simulink library "aerospace"  (R2022a)
settings: Solver=ode45  StartTime=0.0  StopTime=10.0  RelTol=1e-3
undefined symbols (not defined in the file or in its folder): __PRM__SERIALIZED__DATA__, BlockKeywords, convert, Math_Operations_Reshape_convert, Math_Operations_Reshape_reshape, pow
libraries: $bdroot x14
(part 1 of 2)
settings Model: Creator=The MathWorks, Inc.  LastModifiedBy=The MathWorks, Inc.
settings SolverCC: AlgebraicLoopSolver=TrustRegion
settings DataIOCC: LimitDataPoints=on  SaveFormat=Array  SignalLoggingSaveFormat=ModelDataLogs  ReturnWorkspaceOutputs=off
settings OptimizationCC: BlockReduction=off  BooleanDataType=off  ExpressionDepthLimit=2147483647  LifeSpan=inf
settings DebuggingCC: SaveWithParameterizedLinksMsg=none  SignalResolutionControl=TryResolveAllWithWarning  MultiTaskCondExecSysMsg=none  UnconnectedInputMsg=warning  UnconnectedOutputMsg=warning  UnconnectedLineMsg=warning  StateNameClashWarn=warning  SFUnexpectedBacktrackingDiag=warning  SFNoUnconditionalDefaultTransitionDiag=warning  SFExecutionAtInitializationDiag=none  SFMachineParentedDataDiag=warning  ArithmeticOperatorsInVariantConditions=warning
settings HardwareCC: ProdBitPerPointer=32  ProdBitPerSizeT=32  ProdBitPerPtrDiffT=32  ProdLargestAtomicFloat=None  ProdIntDivRoundTo=Undefined  ProdEndianess=Unspecified  ProdWordSize=32  ProdHWDeviceType=32-bit Generic  TargetUnknown=on
settings ModelReferenceCC: PropagateSignalLabelsOutOfModel=off
settings SFSimCC: SimUseLocalCustomCode=off  CustomCodeUndefinedFunction=UseInterfaceOnly
settings RTWCC: RTWUseLocalCustomCode=off
settings CodeAppCC: StateflowObjectComments=on
settings GRTTargetCC: TargetLangStandard=C89/C90 (ANSI)
settings ConfigComp: CovMetricSettings=d  CovSaveCumulativeToWorkspaceVar=on  CovSaveSingleToWorkspaceVar=on  CovExternalEMLEnable=off

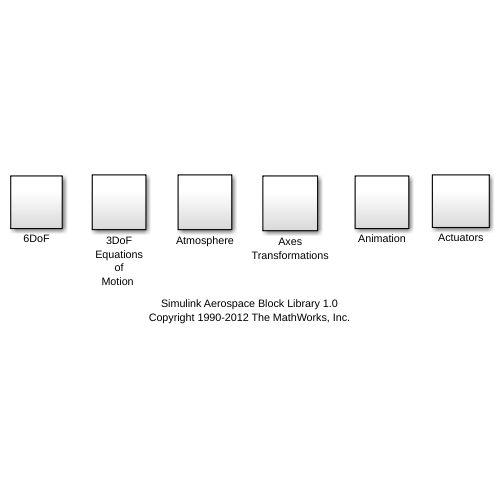
[thumbnail: Simulink's stored preview of the top-level diagram]
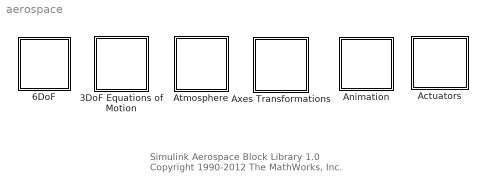
== system aerospace ==
  note: Simulink Aerospace Block Library 1.0
      | Copyright 1990-2012 The MathWorks, Inc.
  "3DoF Equations of Motion " : Subsystem
  6DoF : Subsystem
  Actuators : Subsystem
  Animation : Subsystem
  Atmosphere : Subsystem
  Axes Transformations : Subsystem

== system aerospace/3DoF Equations of Motion  ==
  " Equations of Motion (Body Axes)" : Subsystem  mask(3 DOF equations of motion){v_ini=100, theta_ini=0, alpha_ini=0, q_ini=0, pos_ini=[0 0], mass=1, Iyy=1, g=9.81}
      mask prompts: v_ini "Initial velocity [m/s]:"; theta_ini "Initial body attitude [rad]:"; alpha_ini "Initial incidence [rad]:"; q_ini "Initial body rotation rate [rad/sec]:"; pos_ini "Initial position (x z) [m]:"; mass "Mass [Kg]:"; Iyy "Inertia [Kg.m^2]:"; g "Acceleration due to gravity [m/s/s]:"
      mask help: Integrates the 3 degrees of freedom equations of motion to determine body position, velocity, attitude and related values.
      mask init:
      | U0 = v_ini*cos(alpha_ini);
      | w0 = v_ini*sin(alpha_ini);
      mask Help:
      | <p>This block models the 3 degrees of freedom equations of motion to determine body position, velocity, attitude and other related values.</p>
      | 
      | <p>A 3-down configuration for the body coordinates ( X axis pointing toward nose of body, and  Z axis pointing towards earth) is used in this block.</p>
      | 
      | <p>Gravitational force on the body is already accounted for in this block.</p>
      | 
      | <p>Some block outputs contain more than one signal as described below.</p>
      | 
      | <p><H4>Block  Inputs</H4>
      | <ul>
      |     <li>Forces on the body in X direction - Fx ( N )</li>
      |     <li>Forces on the body in Z direction - Fz ( N ) </li>
      |     <li>Moments on the body along Y direction - M ( N-m )</li>
      | </ul>
      | </p>
      | <p><H4>Block Outputs</H4>
      | <ul>
      |     <li>Pitch angle - Attitude ( radians )</li>
      |     <li>Pitch rate - q ( radians/sec )</li>
      |     <li>Pitch acceleration - qdot ( radians/sec^2 )</li>
      | </ul>
      | </p>
      | <p><H4>Block Vector Output - Xe, Ze </H4>
      | <ul>
      |     <li>Position in X direction in Earth coordinates - Xe ( m )</li>
      |     <li>Position in Z direction in Earth coordinates - Ze ( m )</li>
      | </ul>
      | </p>
      | <p><H4>Block Vector Output - U,w </H4>
      | <ul>
      |     <li>Translational velocity in X direction - U ( m/sec )</li>
      |     <li>Translational velocity in Z direction - w ( m/sec )</li>
      | </ul>
      | </p>
      | <p><H4>Block Vector Output - Ax, Az </H4>
      | <ul>
      |     <li>Acceleration in X direction due to body forces - Ax ( m/sec^2 )</li>
      |     <li>Acceleration in Z direction due to body forces - Az ( m/sec^2 )</li>
      | </ul>
      | </p>
  Incidence & Airspeed : Subsystem  mask(Incidence and Airspeed){}
      mask help: Calculates the angle between the body and the velocity vector (incidence) and the velocity magnitude from the components in body axes (U,w).
      mask Help:
      | <p>This block calculates the angle between the body and the velocity vector (incidence) and the velocity magnitude (airspeed) from the velocity components in body axes (U,w).</p>
      | 
      | <p> A 3-down configuration ( X axis pointing toward nose of body, and  Z axis pointing towards earth) is used in this block.</p>
      | 
      | <p>The block input contains more than one signal as described below.</p>
      | 
      | <p><H4>Block Vector  Input - U,w</H4>
      | <ul>
      |     <li>Translational velocity in X direction - U</li>
      |     <li>Translational velocity in Z direction - w</li>
      | </ul>
      | </p>
      | <p><H4>Block Outputs</H4>
      | <ul>
      |     <li>Incidence angle - alpha (radians)</li>
      |     <li>Airspeed - V</li>
      | </ul>
      | </p>

== system aerospace/6DoF ==
  Equations of Motion (Configurable Subsystem) : Subsystem  Variant=on  VariantControlMode=label  LabelModeActiveChoice=Euler Angles
      settings: AttributesFormatString=%<BlockChoice>
  Euler Angles : Subsystem  mask(6DoF Equations of Motion){xme_0=[0 0 0], Vm_0=[0 0 0], eul_0=[0 0 0], pm_0=[0 0 0], Mass=1.0, Inertia=eye(3)}
      mask prompts: xme_0 "Initial position in inertial axes [Xe,Ye,Ze]:"; Vm_0 "Initial velocity in body axes [U,v,w]:"; eul_0 "Initial Euler orientation [roll, pitch, yaw]:"; pm_0 "Initial body rotation rates [p,q,r]:"; Inertia "Inertia matrix:"
      mask help: Integrates the 6 degrees of freedom equations of motion using an euler angle representation for the orientation of the body in space.
      mask Help:
      | <p>This block models a 6 degrees of freedom equations of motion for a rigid body using an euler angle representation.</p>
      | 
      | <pThe block inputs and outputs contain more than one signal as described below.</p>
      | 
      | <p><H4>Block Vector  Input - Forces X Y Z</H4>
      | <ul>
      |     <li>Forces on the body in X direction - X </li>
      |     <li>Forces on the body in Y direction - Y </li>
      |     <li>Forces on the body in Z direction - Z </li>
      | </ul>
      | </p>
      | <p><H4>Block Vector  Input - Moments L M N</H4>
      | <ul>
      |     <li>Moments on the body along X direction - L </li>
      |     <li>Moments on the body along Y direction - M </li>
      |     <li>Moments on the body along Z direction - N </li>
      | </ul>
      | </p>
      | <p><H4>Block Vector Output - Ve </H4>
      | <ul>
      |     <li>Translational velocity in X direction in Inertial coordinates </li>
      |     <li>Translational velocity in Y direction in Inertial coordinates </li>
      |     <li>Translational velocity in Z direction in Inertial coordinates </li>
      | </ul>
      | </p>
      | <p><H4>Block Vector Output - Xe </H4>
      | <ul>
      |     <li>Position in X direction in Inertial coordinates - Xe </li>
      |     <li>Position in Y direction in Inertial coordinates - Ye </li>
      |     <li>Position in Z direction in Inertial coordinates - Ze </li>
      | </ul>
      | </p>
      | <p><H4>Block Vector Output - Euler </H4>
      | <ul>
      |     <li>Phi ( radians )</li>
      |     <li>Theta ( radians )</li>
      |     <li>Psi ( radians )</li>
      | </ul>
      | </p>
      | <p><H4>Block Vector Output - DMC </H4>
      | <ul>
      |     <li>3x3 Directional Cosine Matrix</li>
      | </ul>
      | </p>
      | <p><H4>Block Vector Output - Vb</H4>
      | <ul>
      |     <li>Translational velocity in X direction in Body coordinates </li>
      |     <li>Translational velocity in Y direction in Body coordinates </li>
      |     <li>Translational velocity in Z direction in Body coordinates </li>
      | </ul>
      | </p>
      | <p><H4>Block Vector Output - p, q, r</H4>
      | <ul>
      |     <li>Roll rate - p ( radians/sec )</li>
      |     <li>Pitch rate - q ( radians/sec )</li>
      |     <li>Yaw rate - r ( radians/sec )</li>
      | </ul>
      | </p>
      | <p><H4>Block Vector Output - pdot, qdot, rdot</H4>
      | <ul>
      |     <li>Roll acceleration - pdot ( radians/sec^2 )</li>
      |     <li>Pitch acceleration - qdot ( radians/sec^2 )</li>
      |     <li>Yaw acceleration - rdot ( radians/sec^2 )</li>
      | </ul>
      | </p>
      mask Display: disp('Euler\nAngles')
  Quaternions : Subsystem  mask(6DoF Equations of Motion){xme_0=[0 0 0], Vm_0=[0 0 0], eul_0=[0 0 0], pm_0=[0 0 0], Mass=1.0, Inertia=eye(3)}
      mask prompts: xme_0 "Initial position in inertial axes [Xe,Ye,Ze]:"; Vm_0 "Initial velocity in body axes [U,v,w]:"; eul_0 "Initial Euler orientation [roll, pitch, yaw]:"; pm_0 "Initial body rotation rates [p,q,r]:"; Inertia "Inertia matrix:"
      mask help: Integrates the 6 degrees of freedom equations of motion using a quaternion representation for the orientation of the body in space.
      mask init:
      | %%% factor used for quaternion calculation
      | k_quat=100;
      | 
      | %%% initial orientation of platform
      | ph=eul_0(1);
      | th=eul_0(2);
      | ps=eul_0(3);
      | e0_0 = cos(0.5*ps)*cos(0.5*th)*cos(0.5*ph) +sin(0.5*ps)*sin(0.5*th)*sin(0.5*ph);
      | e1_0 = cos(0.5*ps)*cos(0.5*th)*sin(0.5*ph) - sin(0.5*ps)*sin(0.5*th)*cos(0.5*ph);
      | e2_0 = cos(0.5*ps)*sin(0.5*th)*cos(0.5*ph) +sin(0.5*ps)*cos(0.5*th)*sin(0.5*ph);
      | e3_0 =-cos(0.5*ps)*sin(0.5*th)*sin(0.5*ph) +sin(0.5*ps)*cos(0.5*th)*cos(0.5*ph);
      mask Help:
      | <p>This block models a 6 degrees of freedom equations of motion for a rigid body using a quaternion representation.</p>
      | 
      | <pThe block inputs and outputs contain more than one signal as described below.</p>
      | 
      | <p><H4>Block Vector  Input - Forces X Y Z</H4>
      | <ul>
      |     <li>Forces on the body in X direction - X </li>
      |     <li>Forces on the body in Y direction - Y </li>
      |     <li>Forces on the body in Z direction - Z </li>
      | </ul>
      | </p>
      | <p><H4>Block Vector  Input - Moments L M N</H4>
      | <ul>
      |     <li>Moments on the body along X direction - L </li>
      |     <li>Moments on the body along Y direction - M </li>
      |     <li>Moments on the body along Z direction - N </li>
      | </ul>
      | </p>
      | <p><H4>Block Vector Output - Ve </H4>
      | <ul>
      |     <li>Translational velocity in X direction in Inertial coordinates </li>
      |     <li>Translational velocity in Y direction in Inertial coordinates </li>
      |     <li>Translational velocity in Z direction in Inertial coordinates </li>
      | </ul>
      | </p>
      | <p><H4>Block Vector Output - Xe </H4>
      | <ul>
      |     <li>Position in X direction in Inertial coordinates - Xe </li>
      |     <li>Position in Y direction in Inertial coordinates - Ye </li>
      |     <li>Position in Z direction in Inertial coordinates - Ze </li>
      | </ul>
      | </p>
      | <p><H4>Block Vector Output - Euler </H4>
      | <ul>
      |     <li>Phi ( radians )</li>
      |     <li>Theta ( radians )</li>
      |     <li>Psi ( radians )</li>
      | </ul>
      | </p>
      | <p><H4>Block Vector Output - DMC </H4>
      | <ul>
      |     <li>3x3 Directional Cosine Matrix</li>
      | </ul>
      | </p>
      | <p><H4>Block Vector Output - Vb</H4>
      | <ul>
      |     <li>Translational velocity in X direction in Body coordinates </li>
      |     <li>Translational velocity in Y direction in Body coordinates </li>
      |     <li>Translational velocity in Z direction in Body coordinates </li>
      | </ul>
      | </p>
      | <p><H4>Block Vector Output - p, q, r</H4>
      | <ul>
      |     <li>Roll rate - p ( radians/sec )</li>
      |     <li>Pitch rate - q ( radians/sec )</li>
      |     <li>Yaw rate - r ( radians/sec )</li>
      | </ul>
      | </p>
      | <p><H4>Block Vector Output - pdot, qdot, rdot</H4>
      | <ul>
      |     <li>Roll acceleration - pdot ( radians/sec^2 )</li>
      |     <li>Pitch acceleration - qdot ( radians/sec^2 )</li>
      |     <li>Yaw acceleration - rdot ( radians/sec^2 )</li>
      | </ul>
      | </p>
      mask Display: disp('Quaternions')

== system aerospace/Actuators ==
  2nd Order Non-linear Actuator : Subsystem  mask(Nonlinear 2nd order actuator model){wn_fin=150, z_fin=0.7, fin_max=20*pi/180, fin_min=-20*pi/180, fin_maxrate=500*pi/180, fin_act_0=0}
      mask prompts: wn_fin "Natural frequency:"; z_fin "Damping ratio:"; fin_max "Maximum deflection:"; fin_min "Minimum deflection:"; fin_maxrate "Maximum rate:"; fin_act_0 "Initial position:"
      mask help:
      | Implement a second-order actuator model with saturation and rate limits, where Ac_dem is the demanded actuator position and Ac_ac is the actual actuator position.
      |
      | Input, output, minimum deflection, maximum deflection, and initial position are in the same position units defined by the input signal.  Maximum rate has the units of position/seconds.
      mask Help:
      | <p>This block contains a model of a second order non-linear actuator.  In addition to setting actuator initial position, damping ratio and natural frequency, block parameters allow fin deflection maximum and minimum limits to be set and a rate limit to be set for the actuator.</p>
      | 
      | <p><H4>Block Input</H4>
      | <ul>
      | <li>Commanded actuator position</li>
      | </ul>
      | </p>
      | 
      | <p><H4>Block Output</H4>
      | <ul>
      | <li>Actual actuator position</li>
      | </ul>
      | </p>
  2nd Order linear Actuator : Subsystem  mask(Linear 2nd order actuator model.){wn_fin=150, z_fin=0.7, fin_act_0=0}
      mask prompts: wn_fin "Natural frequency:"; z_fin "Damping ratio:"; fin_act_0 "Initial position:"
      mask help:
      | Implement a second-order actuator model where Ac_dem is the demanded actuator position and Ac_ac is the actual actuator position.
      |
      | Input, output, and initial position are in the same position units defined by the input signal.
      mask Help:
      | <p>This block contains a model of a second order linear actuator.  Block parameters allow initial position, damping ratio and natural frequency to be set for the  actuator.</p>
      | 
      | <p><H4>Block Input</H4>
      | <ul>
      | <li>Commanded actuator position</li>
      | </ul>
      | </p>
      | 
      | <p><H4>Block Output</H4>
      | <ul>
      | <li>Actual actuator position</li>
      | </ul>
      | </p>

== system aerospace/Animation ==
  3DoF Animation : Subsystem  mask(3DoF Animation){u1=[0 5000 -2000 2000 -5050 -3050], u2=0.05, u3=1, u5=Fixed position, u6=[2000 500 -3150], u7=10, u8=on}
      mask prompts: u1 "Axes limits [xmin xmax ymin ymax zmin zmax]:"; u2 "Time interval between updates:"; u3 "Size of craft displayed:"; u5 "Enter view:"; u6 "Position of camera [xc yc zc]:"; u7 "View angle:"; u8 "Enable animation"
      mask help:
      | Create a 3-D animated view of a three-degrees-of-freedom craft and its target, where X and Z target position (TargetPos), X and Z craft position (Xe,Ze), and craft attitude are inputs.
      |
      | Display parameters are in the same units of length as the input parameters.
      mask init:
      | Config.axes = u1;
      | Config.update = u2;
      | Config.craft = u3;
      | Config.camera_view = u5;
      | Config.camera_pos = u6;
      | Config.view = u7;
      | Config.Animenable = u8;
      mask Help:
      | <p>This block generates a 3 dimensional display of a 3 degrees of freedom trajectory, with the craft's orientation displayed during flight from a viewer position, including a target displayed for the object.  See also: Simulink model 'guidance'.</p>
      | 
      | <p><H4>Block Inputs</H4>
      | <ul>
      | <li>Target position  - [ X, Y, Z ] coordinates
      | <li>[Xe, Ze] - object's range and altitude
      | <li>Attitude - object's pitch angle
      | </ul></p>
      mask TypeOptions u5: Fixed position | Cockpit | Fly alongside
  6DoF Animation : Subsystem  mask(6DoF Animation){u1=[0 4000 -2000 2000 -5000 -3000], u2=0.1, u3=1.0, u4=[4000 0 -5000], u5=Fixed position, u6=[2000 500 -3150], u7=10, u8=on}
      mask prompts: u1 "Axes limits [xmin xmax ymin ymax zmin zmax]:"; u2 "Time interval between updates:"; u3 "Size of craft displayed:"; u4 "Static object position [xp yp zp]:"; u5 "Enter view:"; u6 "Position of camera [xc yc zc]:"; u7 "View angle:"; u8 "Enable animation"
      mask help:
      | Create a 3-D animated view of a six-degrees-of-freedom craft, where X, Y, and Z craft position (Position) and craft Euler angles (Euler) are inputs.
      |
      | Display parameters are in the same units of length as the input parameters.
      mask init:
      | Config.axes = u1;
      | Config.update = u2;
      | Config.craft = u3;
      | Config.target = u4;
      | Config.camera_view = u5;
      | Config.camera_pos = u6;
      | Config.view = u7;
      | Config.Animenable = u8;
      mask Help:
      | <p>This block generates a 3 dimensional display of a simulation trajectory, with the craft orientation displayed during flight</p>
      | 
      | <p>There are two inputs to this block, Position and Euler.  These inputs contain more than one signal as described below.</p>
      | 
      | <p><H4>Block Vector Input - Position</H4>
      | <ul>
      | <li>X Position</li>
      | <li>Y Position</li>
      | <li>Z Position</li>
      | </ul>
      | </p>
      | 
      | <p><H4>Block Vector Input - Euler</H4>
      |     <ul>
      |     <li>Roll Attitude</li>
      |     <li>Pitch Attitude</li>
      |     <li>Yaw Attitude</li>
      |    </ul>
      |    </p>
      mask TypeOptions u5: Fixed position | Cockpit | Fly alongside

== system aerospace/Atmosphere ==
  Atmosphere model : Subsystem  mask(Atmosphere Model){}
      mask help: Compute International Standard Atmosphere (ISA) model for altitudes between 0 Km and 20 Km.
      mask init:
      | g=9.80665; % m/s
      | gamma = 1.4;
      | R = 287.0531; %J/Kg/K
      | L = 0.0065; % K/m
      | h_trop = 11000; % m
      | rho0 = 1.225; %Kg/m^3
      | P0 = 101325; % Pa
      | T0 = 288.15; % K
      mask Help:
      | <p>This block contains the International Standard Atmosphere (ISA) model for altitudes between 0 and 20 Km.  If the height input is greater than 20 Km, the height will be limited to 20 Km.</p>
      | 
      | <p><H4>Block Input</H4>
      | <ul>
      |     <li>Height - Altitude in meters</li>
      | </ul>
      | </p>
      | <p><H4>Block Outputs</H4>
      | <ul>
      |     <li>Temperature - in degree Kelvin</li>
      |     <li>Speed of Sound - in meters/second</li>
      |     <li>Air Pressure - in Pascals</li>
      |     <li>Air Density - in kilograms/meter</li>
      | </ul>
      | </p>

== system aerospace/Axes Transformations ==
  3x3 cross product : Subsystem  mask(Cross Product){}
      mask help: Calculates the cross product of two 3x1 vectors.
      mask Help:
      | <p>This block calculates the cross product of two 3x1 vectors, ie.</p>
      | 
      | <ul>C(1) = A(2)*B(3) - A(3)*B(2)</ul>
      | <ul>C(2) = A(3)*B(1) - A(1)*B(3)</ul>
      | <ul>C(3) = A(1)*B(2) - A(2)*B(1)</ul>
      | 
      | <p>The block inputs and output contain more than one signal as described below.</p>
      | 
      | <p><H4>Block Vector Input 1 - A</H4>
      | <ul>
      | <li>A(1)</li>
      | <li>A(2)</li>
      | <li>A(3)</li>
      | </ul>
      | </p>
      | 
      | <p><H4>Block Vector Input 2 - B</H4>
      | <ul>
      | <li>B(1)</li>
      | <li>B(2)</li>
      | <li>B(3)</li>
      | </ul>
      | </p>
      | 
      | <p><H4>Block Vector Output - Cross Product (AxB)</H4>
      | <ul>
      | <li>C(1)</li>
      | <li>C(2)</li>
      | <li>C(3)</li>
      | </ul>
      | </p>
      mask Display: disp('Cross\nProduct')
  Direction Cosine Matrix from Euler Angles : Subsystem  mask(Direction Cosine Matrix){}
      mask help: Determines the 3x3 Direction Cosine Matrix (DCM) from an euler orientation (roll, pitch, yaw). The outputted DCM transforms vectors from inertial axes to body axes.
      mask Help:
      | <p>This block determines the 3x3 Direction Cosine Matrix (DCM) from a 3x1 euler orientation. The outputted DCM transforms vectors from inertial axes to body axes.</p>
      | 
      | <p>The block input and output contain more than one signal as described below.</p>
      | 
      | <p><H4>Block Vector Input - Euler </H4>
      |     <ul>
      |     <li>Roll Attitude</li>
      |     <li>Pitch Attitude</li>
      |     <li>Yaw Attitude</li>
      |    </ul>
      |    </p>
      | 
      | <p><H4>Block Matrix Output - Direction Cosine Matrix </H4>
      |     <ul>
      |    </ul>
      |    </p>
      mask Display: disp('axis')
  Direction Cosine Matrix from quaternions : Subsystem  mask(Direction Cosine Matrix){}
      mask help: Determines the 3x3 Direction Cosine Matrix (DCM) from a 4x1 quaternion orientation vector. The outputted DCM transforms vectors from inertial axes to body axes.
      mask Help:
      | <p>This block determines the 3x3 Direction Cosine Matrix (DCM) from a 4x1 quaternion orientation vector. The outputted DCM transforms vectors from inertial axes to body axes.</p>
      | 
      | <p>The block input and output contain more than one signal as described below.</p>
      | 
      | <p><H4>Block Vector Input - Quaternion</H4>
      | <ul>
      | <li>q0</li>
      | <li>q1</li>
      | <li>q2</li>
      | <li>q3</li>
      | </ul>
      | </p>
      | 
      | <p><H4>Block Matrix Output - Direction Cosine Matrix  </H4>
      |     <ul>
      |    </ul>
      |    </p>
      mask Display: disp('axis')
  Euler angles from quaternions : Subsystem  mask(Euler angles){}
      mask help: Calculates Euler angles (Roll, Pitch, Yaw) from Quaternions (q0,q1,q2,q3)
      mask Help:
      | <p>This block calculates a 3x1 euler orientation vector from a 4x1 quaternion orientation vector.</p>
      | 
      | <p>The block input and output contain more than one signal as described below.</p>
      | 
      | <p><H4>Block Vector Input - Quaternion</H4>
      | <ul>
      | <li>q0</li>
      | <li>q1</li>
      | <li>q2</li>
      | <li>q3</li>
      | </ul>
      | </p>
      | 
      | <p><H4>Block Vector Output - Euler </H4>
      |     <ul>
      |     <li>Roll Attitude</li>
      |     <li>Pitch Attitude</li>
      |     <li>Yaw Attitude</li>
      |    </ul>
      |    </p>
      mask Display: disp('angles')

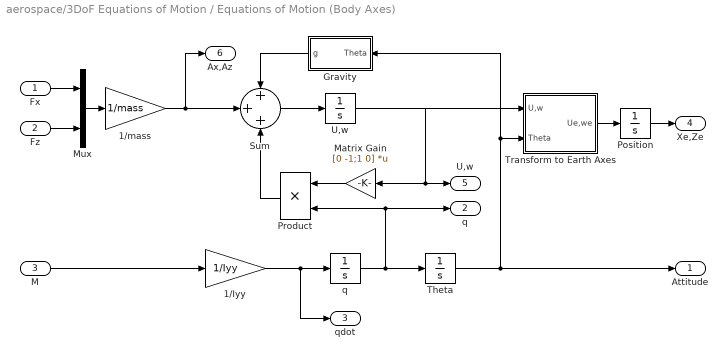
== system aerospace/3DoF Equations of Motion / Equations of Motion (Body Axes) ==
  Fx : Inport
  Fz : Inport  Port=2
  M : Inport  Port=3
  1/Iyy : Gain  Gain=1/Iyy  SaturateOnIntegerOverflow=on  OutDataTypeStr=Inherit: Same as input  ParamDataTypeStr=Inherit: Same as input
  1/mass : Gain  Gain=1/mass  SaturateOnIntegerOverflow=on  OutDataTypeStr=Inherit: Same as input  ParamDataTypeStr=Inherit: Same as input
  Gravity : Subsystem
  Matrix Gain : Gain  Gain=[0 -1;1 0]  Multiplication=Matrix(K*u)  SaturateOnIntegerOverflow=on  OutDataTypeStr=Inherit: Same as input  ParamDataTypeStr=Inherit: Same as input
  Mux : Mux  Inputs=2
  Position : Integrator  InitialCondition=pos_ini
  Product : Product  InputSameDT=on  RndMeth=Zero  SaturateOnIntegerOverflow=on  OutDataTypeStr=Inherit: Same as first input
  Sum : Sum  Inputs=+++  InputSameDT=on  SaturateOnIntegerOverflow=on  OutDataTypeStr=Inherit: Same as first input
  Theta : Integrator  InitialCondition=theta_ini
  Transform to Earth Axes : Subsystem
  U,w : Integrator  InitialCondition=[U0 w0]
  q : Integrator  InitialCondition=q_ini
  Attitude : Outport  InitialOutput=0  VectorParamsAs1DForOutWhenUnconnected=off
  "q " : Outport  Port=2  InitialOutput=0  VectorParamsAs1DForOutWhenUnconnected=off
  qdot : Outport  Port=3  InitialOutput=0  VectorParamsAs1DForOutWhenUnconnected=off
  Xe,Ze : Outport  Port=4  InitialOutput=0  VectorParamsAs1DForOutWhenUnconnected=off
  "U,w " : Outport  Port=5  InitialOutput=0  VectorParamsAs1DForOutWhenUnconnected=off
  Ax,Az : Outport  Port=6  InitialOutput=0  VectorParamsAs1DForOutWhenUnconnected=off
  wires:
  Sum/1 -> U,w/1
  q/1 -> Theta/1, "q "/1, Product/2
  M/1 -> 1/Iyy/1
  1/Iyy/1 -> q/1, qdot/1
  Theta/1 -> Attitude/1, Transform to Earth Axes/2(Theta), Gravity/1(Theta)
  U,w/1 -> Matrix Gain/1, Transform to Earth Axes/1(U,w), "U,w "/1
  Position/1 -> Xe,Ze/1
  Matrix Gain/1 -> Product/1
  Transform to Earth Axes/1(Ue,we) -> Position/1
  Fx/1 -> Mux/1
  Fz/1 -> Mux/2
  Mux/1 -> 1/mass/1
  Product/1 -> Sum/3
  1/mass/1 -> Ax,Az/1, Sum/2
  Gravity/1(g) -> Sum/1

== system aerospace/3DoF Equations of Motion /Incidence & Airspeed ==
  U,w : Inport
  Incidence : Fcn  Expr=atan2(u(2),u(1))
  Velocity : Fcn  Expr=sqrt(u(1)*u(1)+u(2)*u(2))
  Alpha : Outport  InitialOutput=0  VectorParamsAs1DForOutWhenUnconnected=off
  V : Outport  Port=2  InitialOutput=0  VectorParamsAs1DForOutWhenUnconnected=off
  wires:
  Velocity/1 -> V/1
  Incidence/1 -> Alpha/1
  U,w/1 -> Velocity/1, Incidence/1

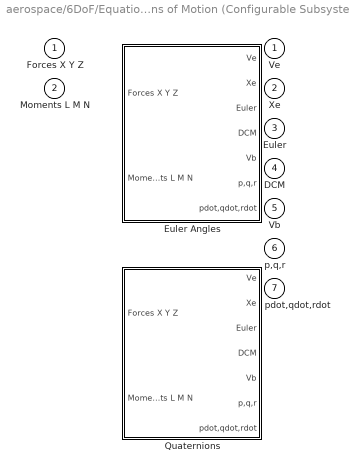
== system aerospace/6DoF/Equations of Motion (Configurable Subsystem) ==
  Forces X Y Z : Inport
  Moments L M N : Inport  Port=2
  Euler Angles : Subsystem  VariantControl=Euler Angles  mask(6DoF Equations of Motion){xme_0=[0 0 0], Vm_0=[0 0 0], eul_0=[0 0 0], pm_0=[0 0 0], Mass=1.0, Inertia=eye(3)}
      mask prompts: xme_0 "Initial position in inertial axes [Xe,Ye,Ze]:"; Vm_0 "Initial velocity in body axes [U,v,w]:"; eul_0 "Initial Euler orientation [roll, pitch, yaw]:"; pm_0 "Initial body rotation rates [p,q,r]:"; Inertia "Inertia matrix:"
      mask help: Integrates the 6 degrees of freedom equations of motion using an euler angle representation for the orientation of the body in space.
      mask Help:
      | <p>This block models a 6 degrees of freedom equations of motion for a rigid body using an euler angle representation.</p>
      | 
      | <pThe block inputs and outputs contain more than one signal as described below.</p>
      | 
      | <p><H4>Block Vector  Input - Forces X Y Z</H4>
      | <ul>
      |     <li>Forces on the body in X direction - X </li>
      |     <li>Forces on the body in Y direction - Y </li>
      |     <li>Forces on the body in Z direction - Z </li>
      | </ul>
      | </p>
      | <p><H4>Block Vector  Input - Moments L M N</H4>
      | <ul>
      |     <li>Moments on the body along X direction - L </li>
      |     <li>Moments on the body along Y direction - M </li>
      |     <li>Moments on the body along Z direction - N </li>
      | </ul>
      | </p>
      | <p><H4>Block Vector Output - Ve </H4>
      | <ul>
      |     <li>Translational velocity in X direction in Inertial coordinates </li>
      |     <li>Translational velocity in Y direction in Inertial coordinates </li>
      |     <li>Translational velocity in Z direction in Inertial coordinates </li>
      | </ul>
      | </p>
      | <p><H4>Block Vector Output - Xe </H4>
      | <ul>
      |     <li>Position in X direction in Inertial coordinates - Xe </li>
      |     <li>Position in Y direction in Inertial coordinates - Ye </li>
      |     <li>Position in Z direction in Inertial coordinates - Ze </li>
      | </ul>
      | </p>
      | <p><H4>Block Vector Output - Euler </H4>
      | <ul>
      |     <li>Phi ( radians )</li>
      |     <li>Theta ( radians )</li>
      |     <li>Psi ( radians )</li>
      | </ul>
      | </p>
      | <p><H4>Block Vector Output - DMC </H4>
      | <ul>
      |     <li>3x3 Directional Cosine Matrix</li>
      | </ul>
      | </p>
      | <p><H4>Block Vector Output - Vb</H4>
      | <ul>
      |     <li>Translational velocity in X direction in Body coordinates </li>
      |     <li>Translational velocity in Y direction in Body coordinates </li>
      |     <li>Translational velocity in Z direction in Body coordinates </li>
      | </ul>
      | </p>
      | <p><H4>Block Vector Output - p, q, r</H4>
      | <ul>
      |     <li>Roll rate - p ( radians/sec )</li>
      |     <li>Pitch rate - q ( radians/sec )</li>
      |     <li>Yaw rate - r ( radians/sec )</li>
      | </ul>
      | </p>
      | <p><H4>Block Vector Output - pdot, qdot, rdot</H4>
      | <ul>
      |     <li>Roll acceleration - pdot ( radians/sec^2 )</li>
      |     <li>Pitch acceleration - qdot ( radians/sec^2 )</li>
      |     <li>Yaw acceleration - rdot ( radians/sec^2 )</li>
      | </ul>
      | </p>
      mask Display: disp('Euler\nAngles')
  Quaternions : Subsystem  VariantControl=Quaternions  mask(6DoF Equations of Motion){xme_0=[0 0 0], Vm_0=[0 0 0], eul_0=[0 0 0], pm_0=[0 0 0], Mass=1.0, Inertia=eye(3)}
      mask prompts: xme_0 "Initial position in inertial axes [Xe,Ye,Ze]:"; Vm_0 "Initial velocity in body axes [U,v,w]:"; eul_0 "Initial Euler orientation [roll, pitch, yaw]:"; pm_0 "Initial body rotation rates [p,q,r]:"; Inertia "Inertia matrix:"
      mask help: Integrates the 6 degrees of freedom equations of motion using a quaternion representation for the orientation of the body in space.
      mask init: same as aerospace/6DoF/Quaternions
      mask Help:
      | <p>This block models a 6 degrees of freedom equations of motion for a rigid body using a quaternion representation.</p>
      | 
      | <pThe block inputs and outputs contain more than one signal as described below.</p>
      | 
      | <p><H4>Block Vector  Input - Forces X Y Z</H4>
      | <ul>
      |     <li>Forces on the body in X direction - X </li>
      |     <li>Forces on the body in Y direction - Y </li>
      |     <li>Forces on the body in Z direction - Z </li>
      | </ul>
      | </p>
      | <p><H4>Block Vector  Input - Moments L M N</H4>
      | <ul>
      |     <li>Moments on the body along X direction - L </li>
      |     <li>Moments on the body along Y direction - M </li>
      |     <li>Moments on the body along Z direction - N </li>
      | </ul>
      | </p>
      | <p><H4>Block Vector Output - Ve </H4>
      | <ul>
      |     <li>Translational velocity in X direction in Inertial coordinates </li>
      |     <li>Translational velocity in Y direction in Inertial coordinates </li>
      |     <li>Translational velocity in Z direction in Inertial coordinates </li>
      | </ul>
      | </p>
      | <p><H4>Block Vector Output - Xe </H4>
      | <ul>
      |     <li>Position in X direction in Inertial coordinates - Xe </li>
      |     <li>Position in Y direction in Inertial coordinates - Ye </li>
      |     <li>Position in Z direction in Inertial coordinates - Ze </li>
      | </ul>
      | </p>
      | <p><H4>Block Vector Output - Euler </H4>
      | <ul>
      |     <li>Phi ( radians )</li>
      |     <li>Theta ( radians )</li>
      |     <li>Psi ( radians )</li>
      | </ul>
      | </p>
      | <p><H4>Block Vector Output - DMC </H4>
      | <ul>
      |     <li>3x3 Directional Cosine Matrix</li>
      | </ul>
      | </p>
      | <p><H4>Block Vector Output - Vb</H4>
      | <ul>
      |     <li>Translational velocity in X direction in Body coordinates </li>
      |     <li>Translational velocity in Y direction in Body coordinates </li>
      |     <li>Translational velocity in Z direction in Body coordinates </li>
      | </ul>
      | </p>
      | <p><H4>Block Vector Output - p, q, r</H4>
      | <ul>
      |     <li>Roll rate - p ( radians/sec )</li>
      |     <li>Pitch rate - q ( radians/sec )</li>
      |     <li>Yaw rate - r ( radians/sec )</li>
      | </ul>
      | </p>
      | <p><H4>Block Vector Output - pdot, qdot, rdot</H4>
      | <ul>
      |     <li>Roll acceleration - pdot ( radians/sec^2 )</li>
      |     <li>Pitch acceleration - qdot ( radians/sec^2 )</li>
      |     <li>Yaw acceleration - rdot ( radians/sec^2 )</li>
      | </ul>
      | </p>
      mask Display: disp('Quaternions')
  Ve : Outport  VectorParamsAs1DForOutWhenUnconnected=off
  Xe : Outport  Port=2  VectorParamsAs1DForOutWhenUnconnected=off
  Euler : Outport  Port=3  VectorParamsAs1DForOutWhenUnconnected=off
  DCM : Outport  Port=4  VectorParamsAs1DForOutWhenUnconnected=off
  Vb : Outport  Port=5  VectorParamsAs1DForOutWhenUnconnected=off
  p,q,r : Outport  Port=6  VectorParamsAs1DForOutWhenUnconnected=off
  pdot,qdot,rdot : Outport  Port=7  VectorParamsAs1DForOutWhenUnconnected=off

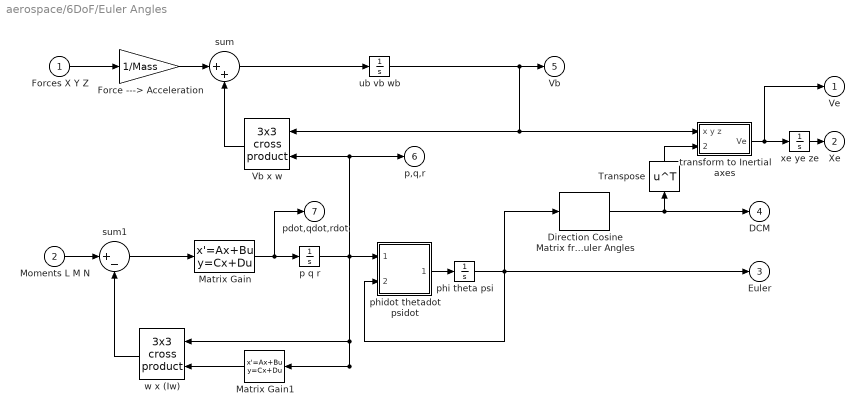
== system aerospace/6DoF/Euler Angles ==
  Forces X Y Z : Inport
  Moments L M N : Inport  Port=2
  Direction Cosine Matrix from Euler Angles : $bdroot/Axes Transformations/Direction Cosine Matrix from Euler Angles
  Force ---> Acceleration : Gain  Gain=1/Mass  SaturateOnIntegerOverflow=on  OutDataTypeStr=Inherit: Same as input  ParamDataTypeStr=Inherit: Same as input
  Matrix Gain : StateSpace  A=[]  B=[]  C=[]  D=K  InitialCondition=0  mask(Matrix Gain){K=inv(Inertia)}
      mask prompts: K "Gain matrix:"
      mask help: Matrix Gain.
      mask Help: Multiplies input vector by entered matrix to produce output vector (y=Au).
      mask Display: disp('Inertia^(-1)')
  Matrix Gain1 : StateSpace  A=[]  B=[]  C=[]  D=K  InitialCondition=0  mask(Matrix Gain){K=Inertia}
      mask prompts: K "Gain matrix:"
      mask help: Matrix Gain.
      mask Help: Multiplies input vector by entered matrix to produce output vector (y=Au).
      mask Display: disp('Inertia')
  Transpose : Math  Operator=transpose  SignedPower=on
  Vb x w : $bdroot/Axes Transformations/3x3 cross product
  p q r : Integrator  InitialCondition=pm_0
  phi theta psi : Integrator  InitialCondition=eul_0
  phidot thetadot psidot : Subsystem
  sum : Sum  Inputs=|++  InputSameDT=on  SaturateOnIntegerOverflow=on  OutDataTypeStr=Inherit: Same as first input
  sum1 : Sum  Inputs=|+-  InputSameDT=on  SaturateOnIntegerOverflow=on  OutDataTypeStr=Inherit: Same as first input
  "transform to Inertial axes " : Subsystem  mask(Vector Transformation){}
      mask Display: disp('L_EB')
  ub vb wb : Integrator  InitialCondition=Vm_0
  w x (Iw) : $bdroot/Axes Transformations/3x3 cross product
  xe ye ze : Integrator  InitialCondition=xme_0
  Ve : Outport  InitialOutput=0  VectorParamsAs1DForOutWhenUnconnected=off
  Xe : Outport  Port=2  InitialOutput=0  VectorParamsAs1DForOutWhenUnconnected=off
  Euler : Outport  Port=3  InitialOutput=0  VectorParamsAs1DForOutWhenUnconnected=off
  DCM : Outport  Port=4  InitialOutput=0  VectorParamsAs1DForOutWhenUnconnected=off
  Vb : Outport  Port=5  InitialOutput=0  VectorParamsAs1DForOutWhenUnconnected=off
  p,q,r : Outport  Port=6  InitialOutput=0  VectorParamsAs1DForOutWhenUnconnected=off
  pdot,qdot,rdot : Outport  Port=7  InitialOutput=0  VectorParamsAs1DForOutWhenUnconnected=off
  wires:
  phidot thetadot psidot/1(phidot thetadot psi) -> phi theta psi/1
  phi theta psi/1 -> Euler/1, phidot thetadot psidot/2(phi theta psi), Direction Cosine Matrix from Euler Angles/1
  ub vb wb/1 -> Vb/1, Vb x w/1, "transform to Inertial axes "/1(x y z)
  sum/1 -> ub vb wb/1
  xe ye ze/1 -> Xe/1
  "transform to Inertial axes "/1(Ve) -> xe ye ze/1, Ve/1
  p q r/1 -> Vb x w/2, p,q,r/1, Matrix Gain1/1, phidot thetadot psidot/1(p q r), w x (Iw)/1
  sum1/1 -> Matrix Gain/1
  Moments L M N/1 -> sum1/1
  Matrix Gain1/1 -> w x (Iw)/2
  w x (Iw)/1 -> sum1/2
  Matrix Gain/1 -> p q r/1, pdot,qdot,rdot/1
  Forces X Y Z/1 -> Force ---> Acceleration/1
  Vb x w/1 -> sum/2
  Force ---> Acceleration/1 -> sum/1
  Direction Cosine Matrix from Euler Angles/1 -> Transpose/1, DCM/1
  Transpose/1 -> "transform to Inertial axes "/2(transform coefficients)

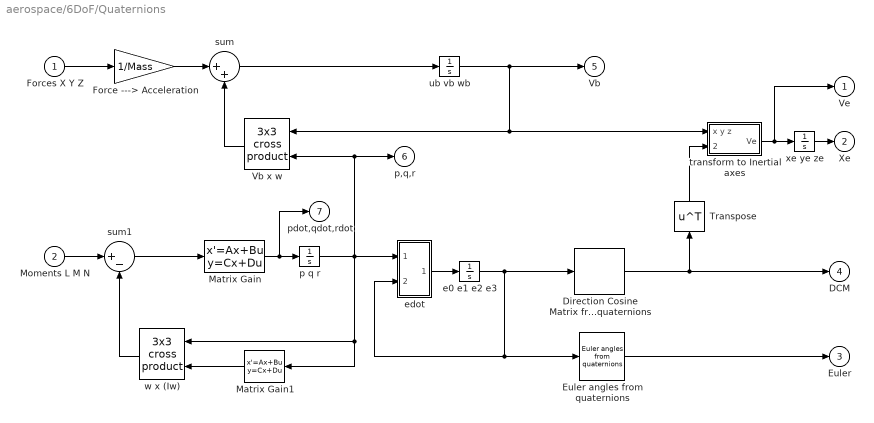
== system aerospace/6DoF/Quaternions ==
  Forces X Y Z : Inport
  Moments L M N : Inport  Port=2
  Direction Cosine Matrix from quaternions : $bdroot/Axes Transformations/Direction Cosine Matrix from quaternions
  Euler angles from quaternions : $bdroot/Axes Transformations/Euler angles from quaternions
  Force ---> Acceleration : Gain  Gain=1/Mass  SaturateOnIntegerOverflow=on  OutDataTypeStr=Inherit: Same as input  ParamDataTypeStr=Inherit: Same as input
  Matrix Gain : StateSpace  A=[]  B=[]  C=[]  D=K  InitialCondition=0  mask(Matrix Gain){K=inv(Inertia)}
      mask prompts: K "Gain matrix:"
      mask help: Matrix Gain.
      mask Help: Multiplies input vector by entered matrix to produce output vector (y=Au).
      mask Display: disp('Inertia^(-1)')
  Matrix Gain1 : StateSpace  A=[]  B=[]  C=[]  D=K  InitialCondition=0  mask(Matrix Gain){K=Inertia}
      mask prompts: K "Gain matrix:"
      mask help: Matrix Gain.
      mask Help: Multiplies input vector by entered matrix to produce output vector (y=Au).
      mask Display: disp('Inertia')
  Transpose : Math  Operator=transpose  SignedPower=on
  Vb x w : $bdroot/Axes Transformations/3x3 cross product
  e0 e1 e2 e3 : Integrator  InitialCondition=[e0_0 e1_0 e2_0 e3_0]
  edot : Subsystem
  p q r : Integrator  InitialCondition=pm_0
  sum : Sum  Inputs=|++  InputSameDT=on  SaturateOnIntegerOverflow=on  OutDataTypeStr=Inherit: Same as first input
  sum1 : Sum  Inputs=|+-  InputSameDT=on  SaturateOnIntegerOverflow=on  OutDataTypeStr=Inherit: Same as first input
  "transform to Inertial axes " : Subsystem  mask(Vector Transformation){}
      mask Display: disp('L_EB')
  ub vb wb : Integrator  InitialCondition=Vm_0
  w x (Iw) : $bdroot/Axes Transformations/3x3 cross product
  xe ye ze : Integrator  InitialCondition=xme_0
  Ve : Outport  InitialOutput=0  VectorParamsAs1DForOutWhenUnconnected=off
  Xe : Outport  Port=2  InitialOutput=0  VectorParamsAs1DForOutWhenUnconnected=off
  Euler : Outport  Port=3  InitialOutput=0  VectorParamsAs1DForOutWhenUnconnected=off
  DCM : Outport  Port=4  InitialOutput=0  VectorParamsAs1DForOutWhenUnconnected=off
  Vb : Outport  Port=5  InitialOutput=0  VectorParamsAs1DForOutWhenUnconnected=off
  p,q,r : Outport  Port=6  InitialOutput=0  VectorParamsAs1DForOutWhenUnconnected=off
  pdot,qdot,rdot : Outport  Port=7  InitialOutput=0  VectorParamsAs1DForOutWhenUnconnected=off
  wires:
  p q r/1 -> edot/1(in_1), Vb x w/2, p,q,r/1, Matrix Gain1/1, w x (Iw)/1
  sum1/1 -> Matrix Gain/1
  Moments L M N/1 -> sum1/1
  Matrix Gain1/1 -> w x (Iw)/2
  w x (Iw)/1 -> sum1/2
  edot/1(out_1) -> e0 e1 e2 e3/1
  e0 e1 e2 e3/1 -> Direction Cosine Matrix from quaternions/1, Euler angles from quaternions/1, edot/2(in_2)
  Euler angles from quaternions/1 -> Euler/1
  Matrix Gain/1 -> p q r/1, pdot,qdot,rdot/1
  Direction Cosine Matrix from quaternions/1 -> Transpose/1, DCM/1
  ub vb wb/1 -> Vb/1, Vb x w/1, "transform to Inertial axes "/1(x y z)
  Forces X Y Z/1 -> Force ---> Acceleration/1
  Vb x w/1 -> sum/2
  sum/1 -> ub vb wb/1
  Force ---> Acceleration/1 -> sum/1
  xe ye ze/1 -> Xe/1
  "transform to Inertial axes "/1(Ve) -> xe ye ze/1, Ve/1
  Transpose/1 -> "transform to Inertial axes "/2(transform coefficients)

== system aerospace/Actuators/2nd Order Non-linear Actuator ==
  Ac_dem : Inport
  2*zeta * wn : Gain  Gain=2.0 * z_fin* wn_fin  SaturateOnIntegerOverflow=on  OutDataTypeStr=Inherit: Same as input  ParamDataTypeStr=Inherit: Same as input
  Demand limits : Saturate  UpperLimit=fin_max  LowerLimit=fin_min
  Limited Deflection : Integrator  InitialCondition=fin_act_0  LimitOutput=on  UpperSaturationLimit=fin_max  LowerSaturationLimit=fin_min
  Servo rate : Integrator
  Sum2 : Sum  Inputs=|+-  InputSameDT=on  SaturateOnIntegerOverflow=on  OutDataTypeStr=Inherit: Same as first input
  Sum3 : Sum  Inputs=|+-  InputSameDT=on  SaturateOnIntegerOverflow=on  OutDataTypeStr=Inherit: Same as first input
  rate limit*2*zeta/wn : Saturate  UpperLimit=fin_maxrate*2*z_fin/wn_fin  LowerLimit=-fin_maxrate*2*z_fin/wn_fin
  wn^2 : Gain  Gain=wn_fin* wn_fin  SaturateOnIntegerOverflow=on  OutDataTypeStr=Inherit: Same as input  ParamDataTypeStr=Inherit: Same as input
  Ac_ac : Outport  InitialOutput=0  VectorParamsAs1DForOutWhenUnconnected=off
  wires:
  Ac_dem/1 -> Demand limits/1
  Demand limits/1 -> Sum3/1
  rate limit*2*zeta/wn/1 -> wn^2/1
  Sum3/1 -> rate limit*2*zeta/wn/1
  2*zeta * wn/1 -> Sum2/2
  Servo rate/1 -> Limited Deflection/1, 2*zeta * wn/1
  Sum2/1 -> Servo rate/1
  wn^2/1 -> Sum2/1
  Limited Deflection/1 -> Sum3/2, Ac_ac/1

== system aerospace/Actuators/2nd Order linear Actuator ==
  Ac_dem : Inport
  2*zeta * wn : Gain  Gain=2.0 * z_fin* wn_fin  SaturateOnIntegerOverflow=on  OutDataTypeStr=Inherit: Same as input  ParamDataTypeStr=Inherit: Same as input
  Servo Deflection : Integrator  InitialCondition=fin_act_0  UpperSaturationLimit=Inf  LowerSaturationLimit=-Inf
  Servo rate : Integrator
  Sum2 : Sum  Inputs=|+-  InputSameDT=on  SaturateOnIntegerOverflow=on  OutDataTypeStr=Inherit: Same as first input
  Sum3 : Sum  Inputs=|+-  InputSameDT=on  SaturateOnIntegerOverflow=on  OutDataTypeStr=Inherit: Same as first input
  wn^2 : Gain  Gain=wn_fin* wn_fin  SaturateOnIntegerOverflow=on  OutDataTypeStr=Inherit: Same as input  ParamDataTypeStr=Inherit: Same as input
  Ac_ac : Outport  InitialOutput=0  VectorParamsAs1DForOutWhenUnconnected=off
  wires:
  Servo Deflection/1 -> Ac_ac/1, Sum3/2
  wn^2/1 -> Sum2/1
  Sum2/1 -> Servo rate/1
  Servo rate/1 -> 2*zeta * wn/1, Servo Deflection/1
  2*zeta * wn/1 -> Sum2/2
  Ac_dem/1 -> Sum3/1
  Sum3/1 -> wn^2/1

== system aerospace/Animation/3DoF Animation ==
  TargetPos : Inport
  Xe,Ze : Inport  Port=2
  Attitude : Inport  Port=3
  Animation S-Function : S-Function  FunctionName=sanim3dof  Parameters=Config  SFunctionDeploymentMode=off  EnableBusSupport=off
  Mux3 : Mux  Inputs=3
  wires:
  Mux3/1 -> Animation S-Function/1
  TargetPos/1 -> Mux3/3
  Attitude/1 -> Mux3/2
  Xe,Ze/1 -> Mux3/1

== system aerospace/Animation/6DoF Animation ==
  Position : Inport
  Euler : Inport  Port=2
  Animation S-Function : S-Function  FunctionName=sanim  Parameters=Config  SFunctionDeploymentMode=off  EnableBusSupport=off
  Mux3 : Mux  Inputs=2
  wires:
  Euler/1 -> Mux3/2
  Position/1 -> Mux3/1
  Mux3/1 -> Animation S-Function/1

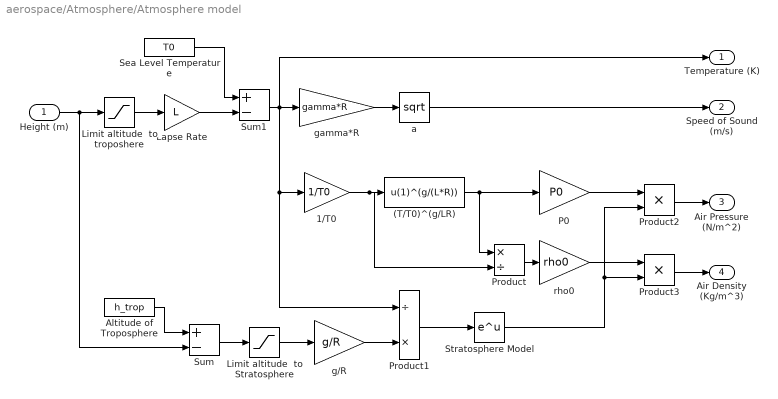
== system aerospace/Atmosphere/Atmosphere model ==
  Height (m) : Inport
  (T/T0)^(g/LR) : Fcn  Expr=u(1)^(g/(L*R))
  1/T0 : Gain  Gain=1/T0  SaturateOnIntegerOverflow=on  OutDataTypeStr=Inherit: Same as input  ParamDataTypeStr=Inherit: Same as input
  Altitude of Troposphere : Constant  Value=h_trop
  Lapse Rate : Gain  Gain=L  SaturateOnIntegerOverflow=on  OutDataTypeStr=Inherit: Same as input  ParamDataTypeStr=Inherit: Same as input
  Limit altitude  to Stratosphere : Saturate  UpperLimit=0  LowerLimit=h_trop-20000
  Limit altitude  to troposhere : Saturate  UpperLimit=h_trop  LowerLimit=0
  P0 : Gain  Gain=P0  SaturateOnIntegerOverflow=on  OutDataTypeStr=Inherit: Same as input  ParamDataTypeStr=Inherit: Same as input
  Product : Product  Inputs=*/  InputSameDT=on  RndMeth=Zero  SaturateOnIntegerOverflow=on  OutDataTypeStr=Inherit: Same as first input
  Product1 : Product  Inputs=/*  InputSameDT=on  RndMeth=Zero  SaturateOnIntegerOverflow=on  OutDataTypeStr=Inherit: Same as first input
  Product2 : Product  InputSameDT=on  RndMeth=Zero  SaturateOnIntegerOverflow=on  OutDataTypeStr=Inherit: Same as first input
  Product3 : Product  InputSameDT=on  RndMeth=Zero  SaturateOnIntegerOverflow=on  OutDataTypeStr=Inherit: Same as first input
  Sea Level Temperature : Constant  Value=T0
  Stratosphere Model : Math  SignedPower=on
  Sum : Sum  Inputs=+-  InputSameDT=on  SaturateOnIntegerOverflow=on  OutDataTypeStr=Inherit: Same as first input
  Sum1 : Sum  Inputs=+-  InputSameDT=on  SaturateOnIntegerOverflow=on  OutDataTypeStr=Inherit: Same as first input
  a : Math  Operator=sqrt  SignedPower=on
  g/R : Gain  Gain=g/R  SaturateOnIntegerOverflow=on  OutDataTypeStr=Inherit: Same as input  ParamDataTypeStr=Inherit: Same as input
  gamma*R : Gain  Gain=gamma*R  SaturateOnIntegerOverflow=on  OutDataTypeStr=Inherit: Same as input  ParamDataTypeStr=Inherit: Same as input
  rho0 : Gain  Gain=rho0  SaturateOnIntegerOverflow=on  OutDataTypeStr=Inherit: Same as input  ParamDataTypeStr=Inherit: Same as input
  Temperature (K) : Outport  InitialOutput=0  VectorParamsAs1DForOutWhenUnconnected=off
  "Speed of Sound (m/s) " : Outport  Port=2  InitialOutput=0  VectorParamsAs1DForOutWhenUnconnected=off
  "Air Pressure (N/m^2) " : Outport  Port=3  InitialOutput=0  VectorParamsAs1DForOutWhenUnconnected=off
  Air Density (Kg/m^3) : Outport  Port=4  InitialOutput=0  VectorParamsAs1DForOutWhenUnconnected=off
  wires:
  Height (m)/1 -> Limit altitude  to troposhere/1, Sum/2
  Limit altitude  to troposhere/1 -> Lapse Rate/1
  Product/1 -> rho0/1
  (T/T0)^(g/LR)/1 -> Product/1, P0/1
  1/T0/1 -> Product/2, (T/T0)^(g/LR)/1
  gamma*R/1 -> a/1
  a/1 -> "Speed of Sound (m/s) "/1
  Sum1/1 -> Temperature (K)/1, gamma*R/1, 1/T0/1, Product1/1
  Lapse Rate/1 -> Sum1/2
  Sea Level Temperature/1 -> Sum1/1
  P0/1 -> Product2/1
  Product2/1 -> "Air Pressure (N/m^2) "/1
  rho0/1 -> Product3/1
  Product3/1 -> Air Density (Kg/m^3)/1
  Stratosphere Model/1 -> Product2/2, Product3/2
  g/R/1 -> Product1/2
  Product1/1 -> Stratosphere Model/1
  Altitude of Troposphere/1 -> Sum/1
  Sum/1 -> Limit altitude  to Stratosphere/1
  Limit altitude  to Stratosphere/1 -> g/R/1

== system aerospace/Axes Transformations/3x3 cross product ==
  a(1) a(2) a(3) : Inport
  b(1) b(2) b(3) : Inport  Port=2
  Product : Product  InputSameDT=on  RndMeth=Zero  SaturateOnIntegerOverflow=on  OutDataTypeStr=Inherit: Same as first input
  Product1 : Product  InputSameDT=on  RndMeth=Zero  SaturateOnIntegerOverflow=on  OutDataTypeStr=Inherit: Same as first input
  Selector : Selector  InputPortWidth=3  IndexOptions=Index vector (dialog)  Indices=[2 3 1]  OutputSizes=1
  Selector1 : Selector  InputPortWidth=3  IndexOptions=Index vector (dialog)  Indices=[3 1 2]  OutputSizes=1
  Selector2 : Selector  InputPortWidth=3  IndexOptions=Index vector (dialog)  Indices=[2 3 1]  OutputSizes=1
  Selector3 : Selector  InputPortWidth=3  IndexOptions=Index vector (dialog)  Indices=[3 1 2]  OutputSizes=1
  Sum : Sum  Inputs=+|-  InputSameDT=on  SaturateOnIntegerOverflow=on  OutDataTypeStr=Inherit: Same as first input
  c(1) c(2) c(3) : Outport  InitialOutput=0  VectorParamsAs1DForOutWhenUnconnected=off
  wires:
  Selector3/1 -> Product1/1
  Selector2/1 -> Product1/2
  Product1/1 -> Sum/2
  Selector1/1 -> Product/2
  Product/1 -> Sum/1
  a(1) a(2) a(3)/1 -> Selector3/1, Selector/1
  Selector/1 -> Product/1
  b(1) b(2) b(3)/1 -> Selector2/1, Selector1/1
  Sum/1 -> c(1) c(2) c(3)/1

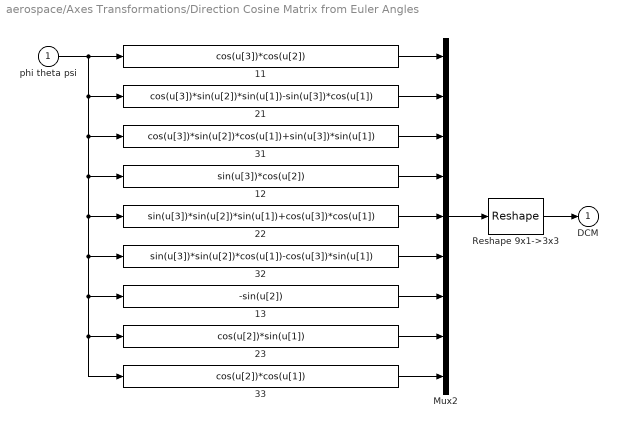
== system aerospace/Axes Transformations/Direction Cosine Matrix from Euler Angles ==
  phi theta psi : Inport
  11 : Fcn  Expr=cos(u[3])*cos(u[2])
  12 : Fcn  Expr=sin(u[3])*cos(u[2])
  13 : Fcn  Expr=-sin(u[2])
  21 : Fcn  Expr=cos(u[3])*sin(u[2])*sin(u[1])-sin(u[3])*cos(u[1])
  22 : Fcn  Expr=sin(u[3])*sin(u[2])*sin(u[1])+cos(u[3])*cos(u[1])
  23 : Fcn  Expr=cos(u[2])*sin(u[1])
  31 : Fcn  Expr=cos(u[3])*sin(u[2])*cos(u[1])+sin(u[3])*sin(u[1])
  32 : Fcn  Expr=sin(u[3])*sin(u[2])*cos(u[1])-cos(u[3])*sin(u[1])
  33 : Fcn  Expr=cos(u[2])*cos(u[1])
  Mux2 : Mux  Inputs=9
  Reshape 9x1->3x3 : Reshape  OutputDimensionality=Customize  OutputDimensions=[3,3]
  DCM : Outport  InitialOutput=0  VectorParamsAs1DForOutWhenUnconnected=off
  wires:
  Reshape 9x1->3x3/1 -> DCM/1
  Mux2/1 -> Reshape 9x1->3x3/1
  11/1 -> Mux2/1
  21/1 -> Mux2/2
  31/1 -> Mux2/3
  12/1 -> Mux2/4
  22/1 -> Mux2/5
  32/1 -> Mux2/6
  13/1 -> Mux2/7
  23/1 -> Mux2/8
  33/1 -> Mux2/9
  phi theta psi/1 -> 11/1, 21/1, 31/1, 12/1, 22/1, 32/1, 13/1, 33/1, 23/1

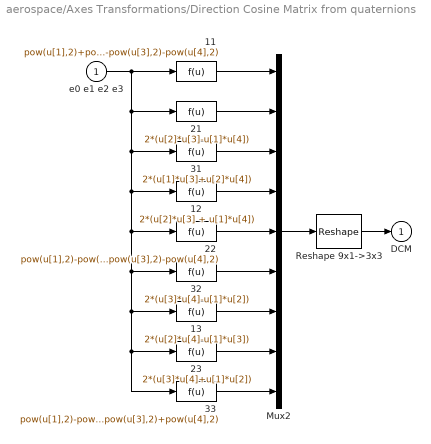
== system aerospace/Axes Transformations/Direction Cosine Matrix from quaternions ==
  e0 e1 e2 e3 : Inport
  11 : Fcn  Expr=pow(u[1],2)+pow(u[2],2)-pow(u[3],2)-pow(u[4],2)
  12 : Fcn  Expr=2*(u[2]*u[3] + u[1]*u[4])
  13 : Fcn  Expr=2*(u[2]*u[4]-u[1]*u[3])
  21 : Fcn  Expr=2*(u[2]*u[3]-u[1]*u[4])
  22 : Fcn  Expr=pow(u[1],2)-pow(u[2],2)+pow(u[3],2)-pow(u[4],2)
  23 : Fcn  Expr=2*(u[3]*u[4]+u[1]*u[2])
  31 : Fcn  Expr=2*(u[1]*u[3]+u[2]*u[4])
  32 : Fcn  Expr=2*(u[3]*u[4]-u[1]*u[2])
  33 : Fcn  Expr=pow(u[1],2)-pow(u[2],2)-pow(u[3],2)+pow(u[4],2)
  Mux2 : Mux  Inputs=9
  Reshape 9x1->3x3 : Reshape  BlockKeywords=__PRM__SERIALIZED__DATA__:convert,2D,Simulink:BlockKeywords:Math_Operations_Reshape_reshape,Simulink:BlockKeywords:Math_Operations_Reshape_convert  OutputDimensionality=Customize  OutputDimensions=[3,3]
  DCM : Outport  InitialOutput=0  VectorParamsAs1DForOutWhenUnconnected=off
  wires:
  Mux2/1 -> Reshape 9x1->3x3/1
  Reshape 9x1->3x3/1 -> DCM/1
  11/1 -> Mux2/1
  21/1 -> Mux2/2
  31/1 -> Mux2/3
  12/1 -> Mux2/4
  22/1 -> Mux2/5
  32/1 -> Mux2/6
  13/1 -> Mux2/7
  23/1 -> Mux2/8
  33/1 -> Mux2/9
  e0 e1 e2 e3/1 -> 11/1, 21/1, 31/1, 12/1, 22/1, 32/1, 13/1, 33/1, 23/1
